simulink model "modele"  (Simulink 7.1)
settings: Solver=ode45  StartTime=0.0  StopTime=2  RelTol=1e-3
undefined symbols (not defined in the file or in its folder): Ac, Ar, Kc, Kr
settings Model: Creator=ahp  LastModifiedBy=ahp

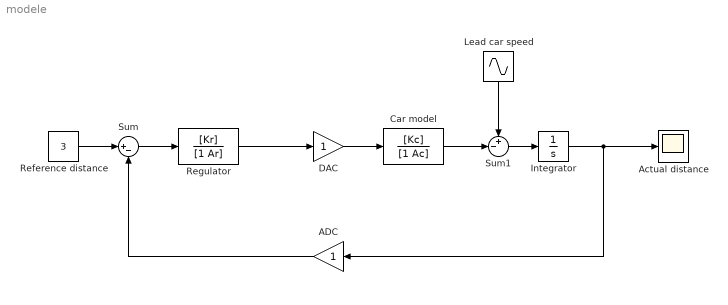
== system modele ==
  ADC : Gain  Orientation=left  ParameterDataType=sfix(16)  ParameterScaling=2^0  OutDataType=sfix(16)  OutScaling=2^0
  Actual distance : Scope
  Car model : TransferFcn  Numerator=[Kc]  Denominator=[1 Ac]
  DAC : Gain  ParameterDataType=sfix(16)  ParameterScaling=2^0  OutDataType=sfix(16)  OutScaling=2^0
  Integrator : Integrator
  Lead car speed : Sin  Orientation=down  SampleTime=0
  Reference distance : Constant  Value=3  OutDataType=sfix(16)  OutScaling=2^0
  Regulator : TransferFcn  Numerator=[Kr]  Denominator=[1 Ar]
  Sum : Sum  Inputs=|+-  OutDataType=sfix(16)  OutScaling=2^0
  Sum1 : Sum  Inputs=+-|  OutDataType=sfix(16)  OutScaling=2^0
  wires:
  Reference distance/1 -> Sum/1
  Sum/1 -> Regulator/1
  Car model/1 -> Sum1/2
  Lead car speed/1 -> Sum1/1
  Sum1/1 -> Integrator/1
  Integrator/1 -> Actual distance/1, ADC/1
  ADC/1 -> Sum/2
  Regulator/1 -> DAC/1
  DAC/1 -> Car model/1
